simulink model "desacoplador_torques"  (R2023b)
settings: Solver=VariableStepAuto  StartTime=0.0  StopTime=10.0  RelTol=1e-3
values from neighbouring files (symbols this model uses):
  beq_nom = bm + bl_nom/r^2    (= 2.19444444444e-05)    [parametros_planta.m]    (also in params_subsistema_mecanico.m; sistema_completo_en_codigo.m)
  g = 9.80665    [controlador_foc_simulink.m]    (also in parametros_planta.m; params_subsistema_mecanico.m; sistema_completo_en_codigo.m)
  kl_nom = m*Lcm + ml_nom*Ll    (= 0.25)    [controlador_foc_simulink.m]    (also in params_subsistema_mecanico.m; sistema_completo_en_codigo.m)
  L_d = 6.6e-3    (= 0.0066)    [controlador_foc_simulink.m]    (also in params_subsistema_electromagnetico.m; sistema_completo_en_codigo.m)
  L_q = 5.8e-3    (= 0.0058)    [controlador_foc_simulink.m]    (also in params_subsistema_electromagnetico.m; sistema_completo_en_codigo.m)
  lambda_m = 0.016    [controlador_foc_simulink.m]    (also in parametros_planta.m; params_subsistema_electromagnetico.m; sistema_completo_en_codigo.m)
  Pp = 3    [controlador_foc_simulink.m]    (also in parametros_planta.m; params_subsistema_electromagnetico.m; sistema_completo_en_codigo.m)
  r = 120.0    (= 120)    [controlador_foc_simulink.m]    (also in parametros_planta.m; params_subsistema_mecanico.m; sistema_completo_en_codigo.m)
settings Model: Creator=Pc  LastModifiedBy=Pc

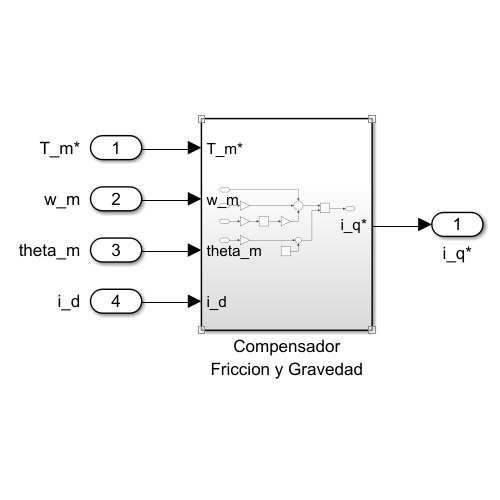
[thumbnail: Simulink's stored preview of the top-level diagram]
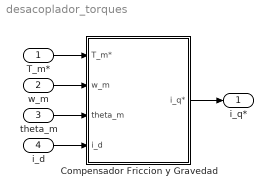
== system desacoplador_torques ==
  T_m* : Inport
  w_m : Inport  Port=2
  theta_m : Inport  Port=3
  i_d : Inport  Port=4
  Compensador Friccion y Gravedad : Subsystem
  i_q* : Outport
  wires:
  T_m*/1 -> Compensador Friccion y Gravedad/1(T_m*)
  w_m/1 -> Compensador Friccion y Gravedad/2(w_m)
  theta_m/1 -> Compensador Friccion y Gravedad/3(theta_m)
  i_d/1 -> Compensador Friccion y Gravedad/4(i_d)
  Compensador Friccion y Gravedad/1(i_q*) -> i_q*/1

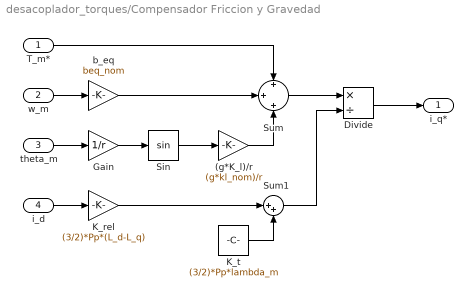
== system desacoplador_torques/Compensador Friccion y Gravedad ==
  T_m* : Inport
  w_m : Inport  Port=2
  theta_m : Inport  Port=3
  i_d : Inport  Port=4
  (g*K_l)/r : Gain  Gain=(g*kl_nom)/r
  Divide : Product  Inputs=*/
  Gain : Gain  Gain=1/r
  K_rel : Gain  Gain=(3/2)*Pp*(L_d-L_q)
  K_t : Constant  Value=(3/2)*Pp*lambda_m
  Sin : Trigonometry
  Sum : Sum  Inputs=+|+|+
  Sum1 : Sum  Inputs=|++
  b_eq : Gain  Gain=beq_nom
  i_q* : Outport
  wires:
  i_d/1 -> K_rel/1
  T_m*/1 -> Sum/1
  Sin/1 -> (g*K_l)/r/1
  K_t/1 -> Sum1/2
  (g*K_l)/r/1 -> Sum/3
  Sum1/1 -> Divide/2
  Gain/1 -> Sin/1
  b_eq/1 -> Sum/2
  K_rel/1 -> Sum1/1
  w_m/1 -> b_eq/1
  Sum/1 -> Divide/1
  Divide/1 -> i_q*/1
  theta_m/1 -> Gain/1
